simulink model "microgrid_y23f_vBackComp"  (R2023b)
settings: Solver=ode23t  StartTime=0.0  StopTime=simu.endTime  FixedStep=0.5  MaxStep=simu.maxStepSize  RelTol=1e-3
undefined symbols (not defined in the file or in its folder): es, mg, pv, wt
libraries: simulink x2
settings Model: Creator=tedbrekken  LastModifiedBy=pldha
settings SolverCC: AlgebraicLoopSolver=TrustRegion
settings DataIOCC: ReturnWorkspaceOutputs=off
settings DebuggingCC: UnconnectedInputMsg=warning  UnconnectedOutputMsg=warning  UnconnectedLineMsg=warning
settings ModelReferenceCC: EnableRefExpFcnMdlSchedulingChecks=on
settings RTWCC: DLArmComputeVersion=19.05

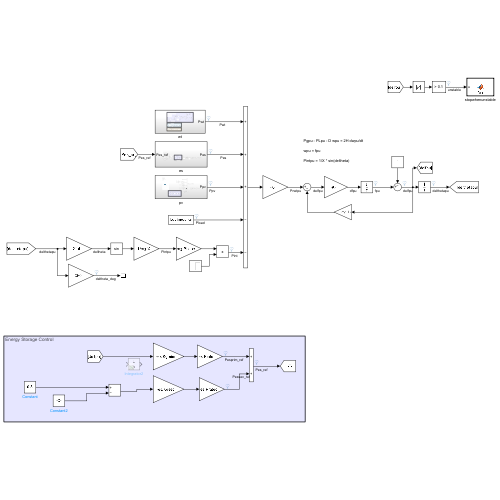
[thumbnail: Simulink's stored preview of the top-level diagram]
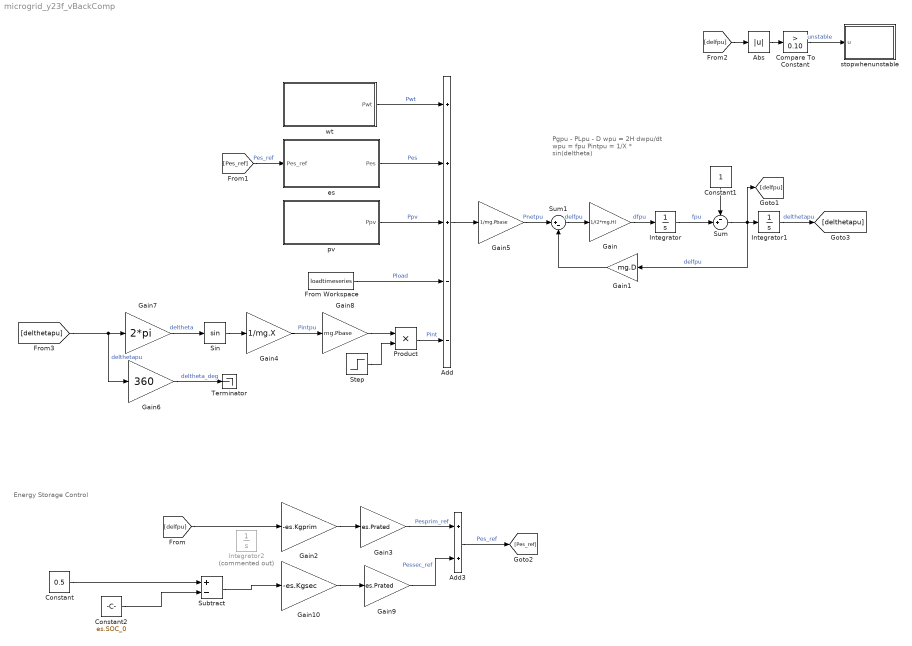
== system microgrid_y23f_vBackComp ==
  note: Energy Storage Control
  note: Pgpu - PLpu - D wpu = 2H dwpu/dt
      |
      | wpu = fpu
      |
      | Pintpu = 1/X * sin(deltheta)
  Abs : Abs  SaturateOnIntegerOverflow=off
  Add : Sum  Inputs=+++--
  Add3 : Sum
  Compare To Constant : simulink/Logic and Bit Operations/Compare To Constant  relop=>  const=0.10  OutDataTypeStr=boolean
  Constant : Constant  Value=0.5
  Constant1 : Constant
  Constant2 : Constant  Value=es.SOC_0
  From Workspace : FromWorkspace  VariableName=loadtimeseries  OutputAfterFinalValue=Setting to zero
  Gain : Gain  Gain=1/(2*mg.H)
  Gain1 : Gain  Gain=mg.D
  Gain10 : Gain  Gain=-es.Kgsec
  Gain2 : Gain  Gain=-es.Kgprim
  Gain3 : Gain  Gain=es.Prated
  Gain4 : Gain  Gain=1/mg.X
  Gain5 : Gain  Gain=1/mg.Pbase
  Gain6 : Gain  Gain=360
  Gain7 : Gain  Gain=2*pi
  Gain8 : Gain  Gain=mg.Pbase
  Gain9 : Gain  Gain=es.Prated
  Integrator : Integrator  InitialCondition=mg.fpu_0
  Integrator1 : Integrator  InitialCondition=mg.fpu_0
  Integrator2 : Integrator  Commented=on
  Product : Product
  Sin : Trigonometry
  Step : Step  Time=12*60*60  After=0  SampleTime=0
  Subtract : Sum  Inputs=+-
  Sum : Sum  Inputs=-+|
  Sum1 : Sum  Inputs=|+-
  Terminator : Terminator
  es : Subsystem
  pv : Subsystem
  stopwhenunstable : MATLAB Function  TreatAsAtomicUnit=on
  wt : Subsystem
  wires:
  [Pes_ref] -> es/1(Pes_ref)  "Pes_ref"
  es/1(Pes) -> Add/2  "Pes"
  wt/1(Pwt) -> Add/1  "Pwt"
  Abs/1 -> Compare To Constant/1
  Compare To Constant/1 -> stopwhenunstable/1(u)  "unstable"
  [delfpu] -> Abs/1
  Add/1 -> Gain5/1
  Gain/1 -> Integrator/1  "dfpu"
  Integrator/1 -> Sum/2  "fpu"
  Gain5/1 -> Sum1/1  "Pnetpu"
  Constant1/1 -> Sum/1
  Sum/1 -> Gain1/1, [delfpu], Integrator1/1  "delfpu"
  Sum1/1 -> Gain/1  "delfpu"
  Gain1/1 -> Sum1/2
  Gain7/1 -> Sin/1  "deltheta"
  Sin/1 -> Gain4/1
  Gain4/1 -> Gain8/1  "Pintpu"
  Gain8/1 -> Product/1
  [delthetapu] -> Gain6/1, Gain7/1  "delthetapu"
  Integrator1/1 -> [delthetapu]  "delthetapu"
  Gain6/1 -> Terminator/1  "deltheta_deg"
  Gain2/1 -> Gain3/1
  Gain3/1 -> Add3/1  "Pesprim_ref"
  Gain9/1 -> Add3/2  "Pessec_ref"
  Add3/1 -> [Pes_ref]  "Pes_ref"
  Gain10/1 -> Gain9/1
  [delfpu] -> Gain2/1
  Product/1 -> Add/5  "Pint"
  Step/1 -> Product/2
  From Workspace/1 -> Add/4  "Pload"
  pv/1(Ppv) -> Add/3  "Ppv"
  Constant/1 -> Subtract/1
  Constant2/1 -> Subtract/2
  Subtract/1 -> Gain10/1

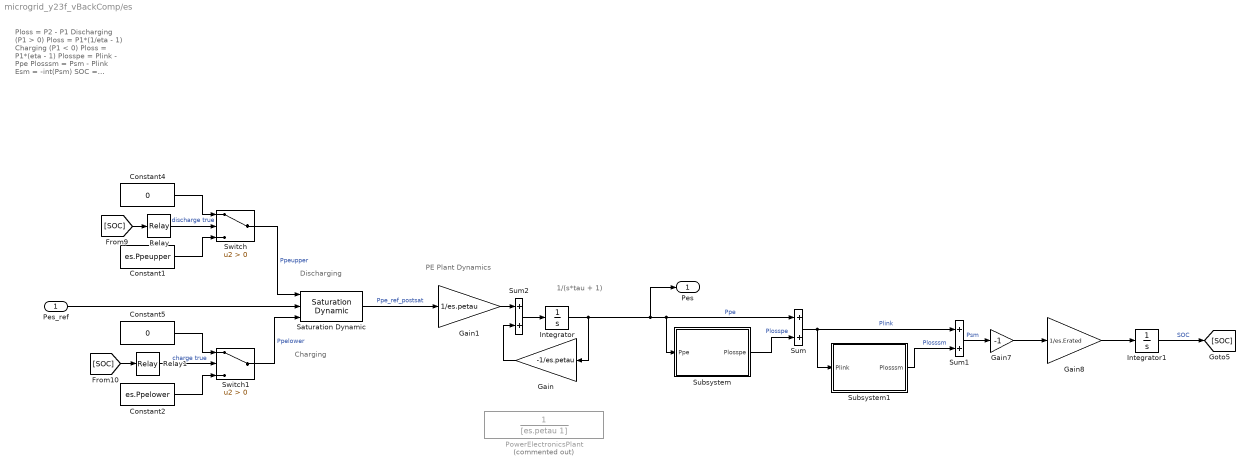
== system microgrid_y23f_vBackComp/es ==
  note: 1/(s*tau + 1)
  note: PE Plant Dynamics
  note: Discharging
  note: Ploss = P2 - P1
      |
      | Discharging (P1 > 0)
      | Ploss = P1*(1/eta - 1)
      |
      | Charging (P1 < 0)
      | Ploss = P1*(eta - 1)
      |
      | Plosspe = Plink - Ppe
      | Plosssm = Psm - Plink
      |
      | Esm = -int(Psm)
      | SOC = Esm/Erated
      |
      | Disharging
      | If Ppe_ref > Ppeupper
      | Ppe = Ppeupper
      |
      | Charging
      | If Ppe_ref < Ppelower
      | Ppe = Ppelower
      |
      | SOC limits
      | if SOC = 0
      | Ppeupper = 0
      | if SOC = 1
      | Ppelower = 0
  note: Charging
  Pes_ref : Inport
  Constant1 : Constant  Value=es.Ppeupper
  Constant2 : Constant  Value=es.Ppelower
  Constant4 : Constant  Value=0
  Constant5 : Constant  Value=0
  Gain : Gain  Gain=-1/es.petau
  Gain1 : Gain  Gain=1/es.petau
  Gain7 : Gain  Gain=-1
  Gain8 : Gain  Gain=1/es.Erated
  Integrator : Integrator  InitialCondition=es.Ppe_0
  Integrator1 : Integrator  InitialCondition=es.SOC_0
  PowerElectronicsPlant : TransferFcn  Commented=on  Denominator=[es.petau 1]
  Relay : Relay  OnSwitchValue=0.01  OffSwitchValue=0  OnOutputValue=0  OffOutputValue=1
  Relay1 : Relay  OnSwitchValue=1  OffSwitchValue=0.99
  Saturation Dynamic : simulink/Discontinuities/Saturation Dynamic  OutMin=[]  OutMax=[]  OutDataTypeStr=Inherit: Same as second input  OutDataType=fixdt(1, 16)  OutScaling=2^-10  DoSatur=off
  Subsystem : Subsystem
  Subsystem1 : Subsystem
  Sum : Sum
  Sum1 : Sum
  Sum2 : Sum
  Switch : Switch  Criteria=u2 > Threshold  SaturateOnIntegerOverflow=off  InputSameDT=off
  Switch1 : Switch  Criteria=u2 > Threshold  SaturateOnIntegerOverflow=off  InputSameDT=off
  Pes : Outport
  wires:
  Subsystem1/1(Plosssm) -> Sum1/2  "Plosssm"
  Relay1/1 -> Switch1/2  "charge true"
  Pes_ref/1 -> Saturation Dynamic/2
  [SOC] -> Relay/1
  Switch/1 -> Saturation Dynamic/1  "Ppeupper"
  Saturation Dynamic/1 -> Gain1/1  "Ppe_ref_postsat"
  Constant5/1 -> Switch1/1
  Switch1/1 -> Saturation Dynamic/3  "Ppelower"
  Gain8/1 -> Integrator1/1
  [SOC] -> Relay1/1
  Subsystem/1(Plosspe) -> Sum/2  "Plosspe"
  Sum1/1 -> Gain7/1  "Psm"
  Constant4/1 -> Switch/1
  Gain7/1 -> Gain8/1
  Constant2/1 -> Switch1/3
  Constant1/1 -> Switch/3
  Relay/1 -> Switch/2  "discharge true"
  Integrator/1 -> Pes/1, Sum/1, Subsystem/1(Ppe), Gain/1  "Ppe"
  Integrator1/1 -> [SOC]  "SOC"
  Sum/1 -> Sum1/1, Subsystem1/1(Plink)  "Plink"
  Sum2/1 -> Integrator/1
  Gain/1 -> Sum2/2
  Gain1/1 -> Sum2/1

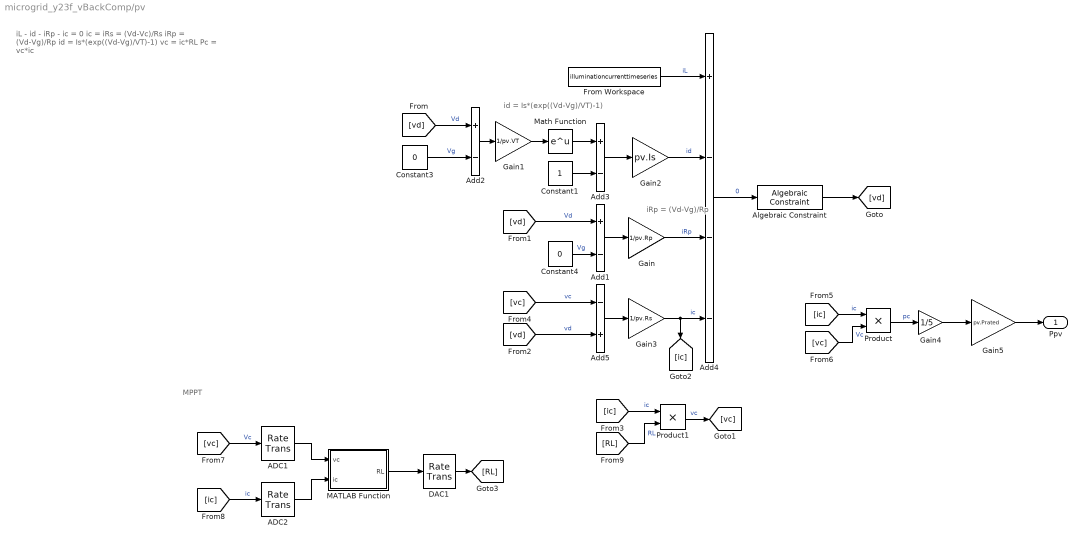
== system microgrid_y23f_vBackComp/pv ==
  note: iRp = (Vd-Vg)/Rp
  note: id = Is*(exp((Vd-Vg)/VT)-1)
  note: MPPT
  note: iL - id - iRp - ic = 0
      |
      | ic = iRs = (Vd-Vc)/Rs
      | iRp = (Vd-Vg)/Rp
      | id = Is*(exp((Vd-Vg)/VT)-1)
      |
      | vc = ic*RL
      |
      | Pc = vc*ic
  ADC1 : RateTransition  OutPortSampleTime=pv.MPPT_sampleTime
  ADC2 : RateTransition  OutPortSampleTime=pv.MPPT_sampleTime
  Add1 : Sum  Inputs=+-
  Add2 : Sum  Inputs=+-
  Add3 : Sum  Inputs=+-
  Add4 : Sum  Inputs=+---
  Add5 : Sum  Inputs=-+
  Algebraic Constraint : AlgebraicConstraint  InitialGuess=0.6
  Constant1 : Constant
  Constant3 : Constant  Value=0
  Constant4 : Constant  Value=0
  DAC1 : RateTransition  OutPortSampleTime=0
  From Workspace : FromWorkspace  VariableName=illuminationcurrenttimeseries  OutputAfterFinalValue=Setting to zero
  Gain : Gain  Gain=1/pv.Rp
  Gain1 : Gain  Gain=1/pv.VT
  Gain2 : Gain  Gain=pv.Is
  Gain3 : Gain  Gain=1/pv.Rs
  Gain4 : Gain  Gain=1/5
  Gain5 : Gain  Gain=pv.Prated
  MATLAB Function : MATLAB Function  TreatAsAtomicUnit=on
  Math Function : Math
  Product : Product
  Product1 : Product
  Ppv : Outport
  wires:
  Gain/1 -> Add4/3  "iRp"
  [vd] -> Add2/1  "Vd"
  Constant3/1 -> Add2/2  "Vg"
  Gain3/1 -> Add4/4, [ic]  "ic"
  [vc] -> Add5/1  "vc"
  Algebraic Constraint/1 -> [vd]
  [ic] -> Product/1  "ic"
  [vc] -> Product/2  "Vc"
  Product/1 -> Gain4/1  "pc"
  [vc] -> ADC1/1  "Vc"
  [ic] -> ADC2/1  "ic"
  DAC1/1 -> [RL]
  ADC1/1 -> MATLAB Function/1(vc)
  ADC2/1 -> MATLAB Function/2(ic)
  MATLAB Function/1(RL) -> DAC1/1
  From Workspace/1 -> Add4/1  "iL"
  Add4/1 -> Algebraic Constraint/1  "0"
  Add2/1 -> Gain1/1
  Gain1/1 -> Math Function/1
  Math Function/1 -> Add3/1
  Constant1/1 -> Add3/2
  Add3/1 -> Gain2/1
  Gain2/1 -> Add4/2  "id"
  [vd] -> Add1/1  "Vd"
  Constant4/1 -> Add1/2  "Vg"
  Add1/1 -> Gain/1
  [vd] -> Add5/2  "vd"
  Add5/1 -> Gain3/1
  [ic] -> Product1/1  "ic"
  [RL] -> Product1/2  "RL"
  Product1/1 -> [vc]  "vc"
  Gain4/1 -> Gain5/1
  Gain5/1 -> Ppv/1

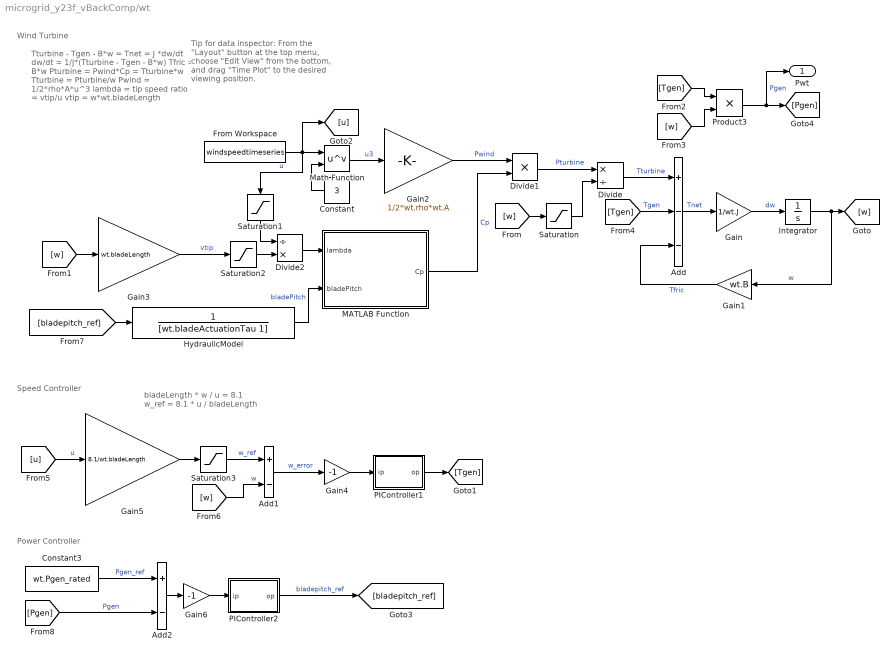
== system microgrid_y23f_vBackComp/wt ==
  note: Wind Turbine
  note: Tturbine - Tgen - B*w = Tnet = J *dw/dt
      | dw/dt = 1/J*(Tturbine - Tgen - B*w)
      |
      | Tfric = B*w
      |
      | Pturbine = Pwind*Cp = Tturbine*w
      | Tturbine = Pturbine/w
      |
      | Pwind = 1/2*rho*A*u^3
      |
      | lambda = tip speed ratio = vtip/u
      | vtip = w*wt.bladeLength
  note: Tip for data inspector: From the "Layout" button at the top menu, choose "Edit View" from the bottom, and drag "Time Plot" to the desired viewing position.
  note: bladeLength * w / u = 8.1
      | w_ref = 8.1 * u / bladeLength
  note: Power Controller
  note: Speed Controller
  Add : Sum  Inputs=+--
  Add1 : Sum  Inputs=+-
  Add2 : Sum  Inputs=+-
  Constant : Constant  Value=3
  Constant3 : Constant  Value=wt.Pgen_rated
  Divide : Product  Inputs=*/
  Divide1 : Product  Inputs=**
  Divide2 : Product  Inputs=/*
  From Workspace : FromWorkspace  VariableName=windspeedtimeseries
  Gain : Gain  Gain=1/wt.J
  Gain1 : Gain  Gain=wt.B
  Gain2 : Gain  Gain=1/2*wt.rho*wt.A
  Gain3 : Gain  Gain=wt.bladeLength
  Gain4 : Gain  Gain=-1
  Gain5 : Gain  Gain=8.1/wt.bladeLength
  Gain6 : Gain  Gain=-1
  HydraulicModel : TransferFcn  Denominator=[wt.bladeActuationTau 1]
  Integrator : Integrator  InitialCondition=wt.w_0
  MATLAB Function : MATLAB Function  TreatAsAtomicUnit=on
  Math Function : Math  Operator=pow
  PIController1 : Subsystem  mask{kp=wt.speedcontroller.kp, ki=wt.speedcontroller.ki, kt=wt.speedcontroller.kt, upperLimit=wt.speedcontroller.upperLimit, lowerLimit=wt.speedcontroller.lowerLimit, int_0=wt.speedcontroller.int_0}
      mask prompts: kp "Proportional gain"; ki "Integral gain"; kt "Windup gain"; upperLimit "Upper limit"; lowerLimit "Lower limit"; int_0 "Initial condition"
  PIController2 : Subsystem  mask{kp=wt.powercontroller.kp, ki=wt.powercontroller.ki, kt=wt.powercontroller.kt, upperLimit=wt.powercontroller.upperLimit, lowerLimit=wt.powercontroller.lowerLimit, int_0=wt.powercontroller.int_0}
      mask prompts: kp "Proportional gain"; ki "Integral gain"; kt "Windup gain"; upperLimit "Upper limit"; lowerLimit "Lower limit"; int_0 "Initial condition"
  Product3 : Product
  Saturation : Saturate  UpperLimit=inf  LowerLimit=1e-3
  Saturation1 : Saturate  UpperLimit=inf  LowerLimit=1e-3
  Saturation2 : Saturate  UpperLimit=inf  LowerLimit=1e-3
  Saturation3 : Saturate  UpperLimit=wt.w_rated  LowerLimit=0
  Pwt : Outport
  wires:
  MATLAB Function/1(Cp) -> Divide1/2  "Cp"
  Add1/1 -> Gain4/1  "w_error"
  [bladepitch_ref] -> HydraulicModel/1
  Math Function/1 -> Gain2/1  "u3"
  HydraulicModel/1 -> MATLAB Function/2(bladePitch)  "bladePitch"
  Product3/1 -> Pwt/1, [Pgen]  "Pgen"
  [w] -> Gain3/1
  Saturation3/1 -> Add1/1  "w_ref"
  Saturation/1 -> Divide/2
  [Pgen] -> Add2/2  "Pgen"
  Gain5/1 -> Saturation3/1
  Saturation1/1 -> Divide2/1
  [w] -> Saturation/1
  PIController2/1(op) -> [bladepitch_ref]  "bladepitch_ref"
  Gain4/1 -> PIController1/1(ip)
  Constant3/1 -> Add2/1  "Pgen_ref"
  Gain6/1 -> PIController2/1(ip)
  From Workspace/1 -> [u], Saturation1/1, Math Function/1  "u"
  Divide/1 -> Add/1  "Tturbine"
  [w] -> Add1/2  "w"
  Constant/1 -> Math Function/2
  [Tgen] -> Add/2  "Tgen"
  Gain1/1 -> Add/3  "Tfric"
  Integrator/1 -> [w], Gain1/1  "w"
  Gain2/1 -> Divide1/1  "Pwind"
  Add/1 -> Gain/1  "Tnet"
  [u] -> Gain5/1  "u"
  PIController1/1(op) -> [Tgen]
  Saturation2/1 -> Divide2/2
  Divide2/1 -> MATLAB Function/1(lambda)
  Gain/1 -> Integrator/1  "dw"
  Gain3/1 -> Saturation2/1  "vtip"
  Add2/1 -> Gain6/1
  [w] -> Product3/2
  [Tgen] -> Product3/1
  Divide1/1 -> Divide/1  "Pturbine"

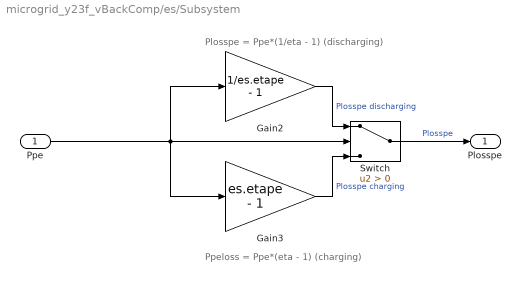
== system microgrid_y23f_vBackComp/es/Subsystem ==
  note: Ppeloss = Ppe*(eta - 1) (charging)
  note: Plosspe = Ppe*(1/eta - 1) (discharging)
  Ppe : Inport
  Gain2 : Gain  Gain=1/es.etape - 1
  Gain3 : Gain  Gain=es.etape - 1
  Switch : Switch  Criteria=u2 > Threshold  SaturateOnIntegerOverflow=off  InputSameDT=off
  Plosspe : Outport
  wires:
  Gain3/1 -> Switch/3  "Plosspe charging"
  Gain2/1 -> Switch/1  "Plosspe discharging"
  Switch/1 -> Plosspe/1  "Plosspe"
  Ppe/1 -> Gain2/1, Gain3/1, Switch/2

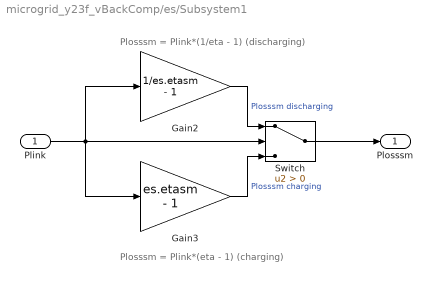
== system microgrid_y23f_vBackComp/es/Subsystem1 ==
  note: Plosssm = Plink*(eta - 1) (charging)
  note: Plosssm = Plink*(1/eta - 1) (discharging)
  Plink : Inport
  Gain2 : Gain  Gain=1/es.etasm - 1
  Gain3 : Gain  Gain=es.etasm - 1
  Switch : Switch  Criteria=u2 > Threshold  SaturateOnIntegerOverflow=off  InputSameDT=off
  Plosssm : Outport
  wires:
  Gain3/1 -> Switch/3  "Plosssm charging"
  Gain2/1 -> Switch/1  "Plosssm discharging"
  Switch/1 -> Plosssm/1
  Plink/1 -> Gain2/1, Gain3/1, Switch/2

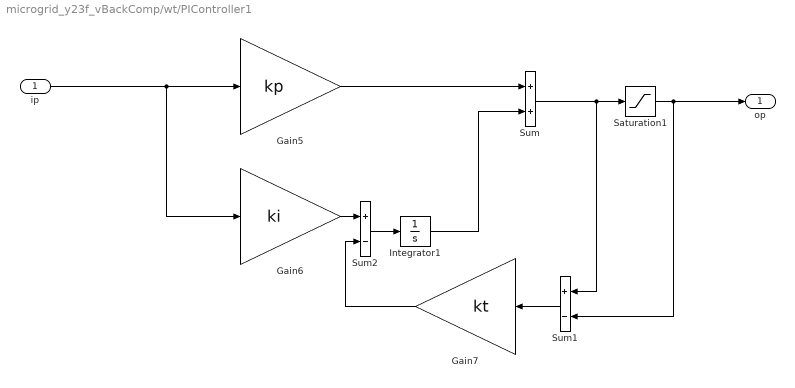
== system microgrid_y23f_vBackComp/wt/PIController1 ==
  ip : Inport
  Gain5 : Gain  Gain=kp
  Gain6 : Gain  Gain=ki
  Gain7 : Gain  Gain=kt
  Integrator1 : Integrator  InitialCondition=int_0
  Saturation1 : Saturate  UpperLimit=upperLimit  LowerLimit=lowerLimit
  Sum : Sum
  Sum1 : Sum  Inputs=+-
  Sum2 : Sum  Inputs=+-
  op : Outport
  wires:
  Sum2/1 -> Integrator1/1
  Integrator1/1 -> Sum/2
  Gain7/1 -> Sum2/2
  Sum1/1 -> Gain7/1
  Gain6/1 -> Sum2/1
  ip/1 -> Gain6/1, Gain5/1
  Saturation1/1 -> op/1, Sum1/2
  Gain5/1 -> Sum/1
  Sum/1 -> Sum1/1, Saturation1/1

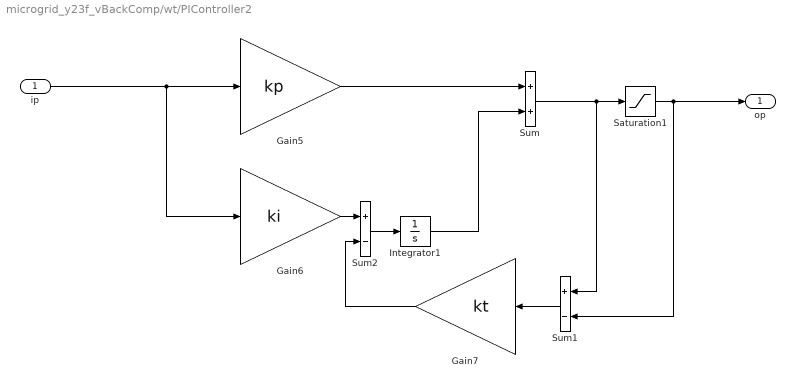
== system microgrid_y23f_vBackComp/wt/PIController2 ==
  ip : Inport
  Gain5 : Gain  Gain=kp
  Gain6 : Gain  Gain=ki
  Gain7 : Gain  Gain=kt
  Integrator1 : Integrator  InitialCondition=int_0
  Saturation1 : Saturate  UpperLimit=upperLimit  LowerLimit=lowerLimit
  Sum : Sum
  Sum1 : Sum  Inputs=+-
  Sum2 : Sum  Inputs=+-
  op : Outport
  wires:
  Sum2/1 -> Integrator1/1
  Integrator1/1 -> Sum/2
  Gain7/1 -> Sum2/2
  Sum1/1 -> Gain7/1
  Gain6/1 -> Sum2/1
  ip/1 -> Gain6/1, Gain5/1
  Saturation1/1 -> op/1, Sum1/2
  Gain5/1 -> Sum/1
  Sum/1 -> Sum1/1, Saturation1/1

== matlab function microgrid_y23f_vBackComp/wt/MATLAB Function ==
  data: lambda input; Cp output; bladePitch input
function Cp = fcn(lambda,bladePitch)

% https://www.mathworks.com/help/physmod/sps/powersys/ref/windturbine.html

c = [...
    0.5176 ...
    116 ...
    0.4 ...
    5 ...
    21 ...
    0.0068];

lambdaai = 1/( 1/(lambda+0.08*bladePitch) - 0.035/(bladePitch^3+1) );

Cp = c(1)*(c(2)/lambdaai-c(3)*bladePitch-c(4))*exp(-c(5)/lambdaai) + c(6)*lambda;

== matlab function microgrid_y23f_vBackComp/pv/MATLAB Function ==
  data: vc input; RL output; ic input
function RL = fcn(vc, ic)
 persistent vcprev icprev dirprev RLprev 
 if isempty(vcprev) 
 vcprev = 0; 
 end 
 if isempty(icprev) 
 icprev = 0; 
 end 
 if isempty(dirprev) 
 dirprev = 1; 
 end 
 if isempty(RLprev) 
 RLprev = 0; 
 end 
 Pc = vc*ic; 
 Pcprev = vcprev*icprev; 
 if Pc > Pcprev 
 dir = dirprev; 
 elseif Pc < Pcprev 
 dir = -dirprev; 
 else 
 dir = 1; 
 end 
 RL = RLprev + dir*0.005; 
 if RL < 0 
 RL = 0; 
 end 
 if RL > 1 
 RL = 1; 
 end

== matlab function microgrid_y23f_vBackComp/stopwhenunstable ==
  data: u input
function fcn(u)

if u == 1
    error('Frequency out of bounds.  Microgrid failed.')
end
